simulink model "Hard_simulink"  (R2014a)
settings: Solver=ode45  StartTime=0.0  StopTime=10.0  RelTol=1e-3
libraries: commdigbbndpm3 x2, commcnvcod2 x2, commchan3 x1, commrandsrc2 x1, commsink2 x1
settings Model: Creator=华联  LastModifiedBy=10575

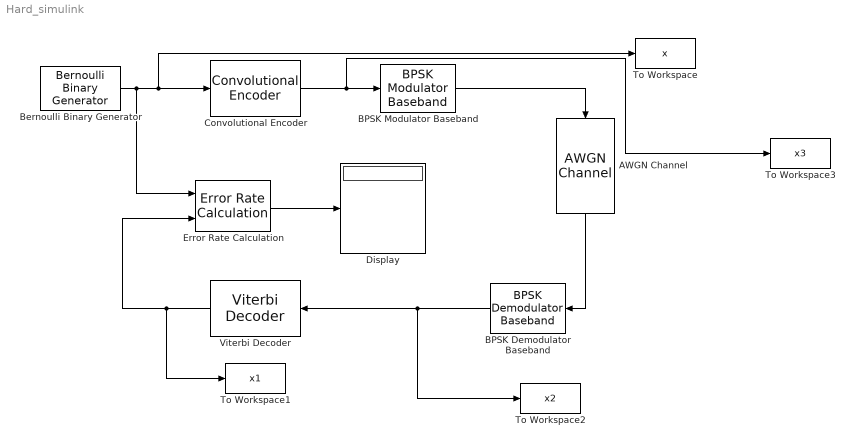
== system Hard_simulink ==
  AWGN Channel : commchan3/AWGN Channel  InputProcessing=Columns as channels (frame based)  seed=67  noiseMode="Signal to noise ratio  (Eb/No)"  EbNodB=10  EsNodB=10  SNRdB=10  bitsPerSym=1  Ps=1  Tsym=1  variance=1
  BPSK Demodulator Baseband : commdigbbndpm3/BPSK Demodulator Baseband  Ph=0  DecType=Hard decision  VarSource=Dialog  Variance=1  outDtype=Inherit via internal rule  derotateFactorWordLen=16
  BPSK Modulator Baseband : commdigbbndpm3/BPSK Modulator Baseband  Ph=0  outDtype=double  outWordLen=16  outUDDataType=sfix(16)  outFracLenMode=Best precision  outFracLen=15
  Bernoulli Binary Generator : commrandsrc2/Bernoulli Binary Generator  P=0.5  seed=61  Ts=1  frameBased=off  sampPerFrame=1  orient=off  outDataType=double
  Convolutional Encoder : commcnvcod2/Convolutional Encoder  trellis=poly2trellis(3, [7 5])  opMode=Continuous  DelayedResetAction=off  hasIniStPort=off  hasFinStPort=off  usePuncVector=off  punctureVector=[1; 1; 0; 1; 0; 1]  reset=Unused parameter value
  Display : Display
  Error Rate Calculation : commsink2/Error Rate Calculation  N=0  st_delay=0  cp_mode=Entire frame  subframe=[]  PMode=Port  WsName=ErrorVec  RsMode2=off  stop=off  numErr=100  maxBits=1e6
  To Workspace : ToWorkspace  VariableName=x  SampleTime=-1
  To Workspace1 : ToWorkspace  VariableName=x1  SampleTime=-1
  To Workspace2 : ToWorkspace  VariableName=x2  SampleTime=-1
  To Workspace3 : ToWorkspace  VariableName=x3  SampleTime=-1
  Viterbi Decoder : commcnvcod2/Viterbi Decoder  trellis=poly2trellis(3, [7 5])  isPunctured=off  punctureVector=[1; 1; 0; 1; 0; 1]  erasures=off  dectype=Hard decision  runSigValErrCheck=off  nsdecb=4  smWordLength=16  tbdepth=34  opmode=Continuous  reset=off  outDataType=Inherit via internal rule  delayedResetAction=off
  wires:
  Bernoulli Binary Generator/1 -> Error Rate Calculation/1, To Workspace/1, Convolutional Encoder/1
  Convolutional Encoder/1 -> To Workspace3/1, BPSK Modulator Baseband/1
  Viterbi Decoder/1 -> To Workspace1/1, Error Rate Calculation/2
  BPSK Demodulator Baseband/1 -> To Workspace2/1, Viterbi Decoder/1
  AWGN Channel/1 -> BPSK Demodulator Baseband/1
  BPSK Modulator Baseband/1 -> AWGN Channel/1
  Error Rate Calculation/1 -> Display/1
